simulink model "lhj_zero_optimize_2018a"  (R2018a)
settings: Solver=FixedStepDiscrete  StartTime=0.0  StopTime=0.2  FixedStep=Ts  RelTol=1e-4
InitFcn:
  | Ts=1e-6;
libraries: powerlib x17, simulink x2
settings Model: ExtModeTrigMode=oneshot  ExtModeArmWhenConnect=off  ExtModeAutoUpdateStatusClock=off  Creator=patrice  LastModifiedBy=chengqian
settings DataIOCC: SaveFormat=Array  SignalLoggingSaveFormat=ModelDataLogs  SignalLoggingName=sigsOut
settings OptimizationCC: BlockReduction=off  BooleanDataType=off  ExpressionDepthLimit=2147483647  InitFltsAndDblsToZero=on  LifeSpan=inf
settings DebuggingCC: SaveWithParameterizedLinksMsg=none  UnderspecifiedInitializationDetection=Classic  MergeDetectMultiDrivingBlocksExec=none  CheckExecutionContextPreStartOutputMsg=on  CheckExecutionContextRuntimeOutputMsg=on  SignalResolutionControl=TryResolveAllWithWarning  MultiTaskDSMMsg=warning  MultiTaskCondExecSysMsg=none  FcnCallInpInsideContextMsg=warning  UnconnectedLineMsg=none  StateNameClashWarn=warning  SFUnexpectedBacktrackingDiag=warning  SFNoUnconditionalDefaultTransitionDiag=warning  SFExecutionAtInitializationDiag=none
settings HardwareCC: ProdBitPerPointer=32  ProdBitPerSizeT=32  ProdBitPerPtrDiffT=32  ProdLargestAtomicFloat=None  ProdIntDivRoundTo=Undefined  ProdEndianess=Unspecified  ProdWordSize=32  ProdHWDeviceType=32-bit Generic  TargetUnknown=on
settings ModelReferenceCC: PropagateSignalLabelsOutOfModel=off
settings RTWCC: TemplateMakefile=grt_unix.tmf
settings CodeAppCC: StateflowObjectComments=on
settings GRTTargetCC: TargetFcnLib=ansi_tfl_tmw.mat  TargetLangStandard=C89/C90 (ANSI)  CombineOutputUpdateFcns=off  GRTInterface=on
settings ConfigComp: CovMetricSettings=dw  CovHtmlReporting=on  CovSaveCumulativeToWorkspaceVar=on  CovSaveSingleToWorkspaceVar=on  CovExternalEMLEnable=off

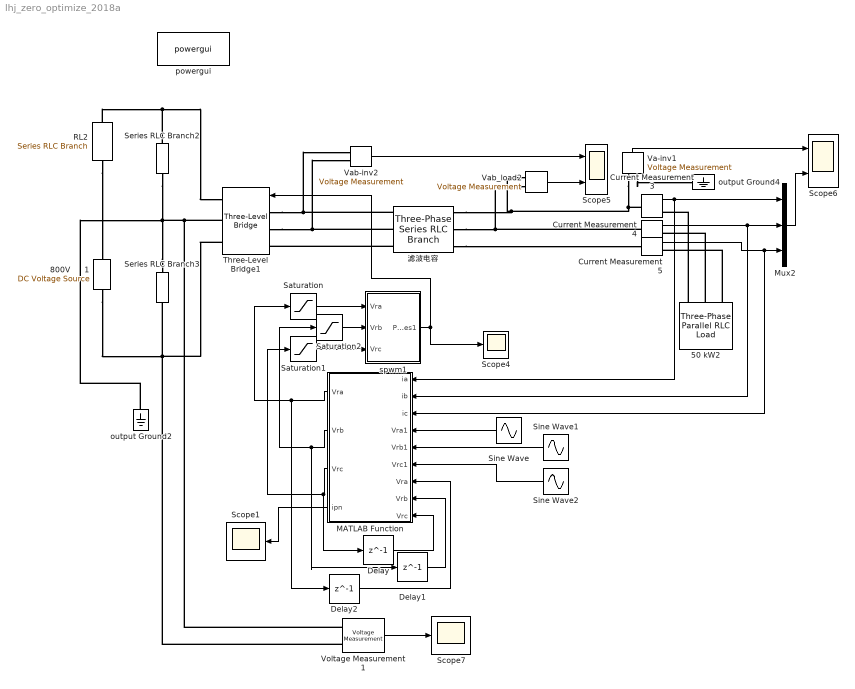
== system lhj_zero_optimize_2018a ==
  " 滤波电容" : powerlib/Elements/Three-Phase Series RLC Branch  LConnTagsString=A|B|C  RConnTagsString=A|B|C  BranchType=L  Resistance=0.1  Inductance=0.02  Capacitance=30e-3  Measurements=None
      settings: SourceProductName=Simscape Electrical
  50 kW2 : powerlib/Elements/Three-Phase Parallel RLC Load  LConnTagsString=A|B|C  Configuration=Y (grounded)  NominalVoltage=650  Vabc=[1e3 1e3 1e3]  Vabcp=[1e3 1e3 1e3]  NominalFrequency=50  UnbalancedPower=off  ActivePower=20000  InductivePower=0  CapacitivePower=0  Pabc=[10e3 9e3 11e3]  QLabc=[100 90 110]  QCabc=[100 90 110]  Pabcp=[10e3 9e3 11e3]  QLabcp=[100 90 110]  QCabcp=[100 90 110]  Measurements=Branch currents  LoadType=constant Z
      settings: SourceProductName=Simscape Electrical
  800V      1 : powerlib/Electrical Sources/DC Voltage Source  Description=source block  Amplitude=800  Measurements=None
      settings: AttributesFormatString=\n  SourceProductName=Simscape Electrical
  Current Measurement3 : powerlib/Measurements/Current Measurement  PhasorSimulation=off  OutputType=Complex  PSBequivalent=0
      settings: SourceProductName=Simscape Electrical
  Current Measurement4 : powerlib/Measurements/Current Measurement  PhasorSimulation=off  OutputType=Complex  PSBequivalent=0
      settings: SourceProductName=Simscape Electrical
  Current Measurement5 : powerlib/Measurements/Current Measurement  PhasorSimulation=off  OutputType=Complex  PSBequivalent=0
      settings: SourceProductName=Simscape Electrical
  Delay : Delay  DelayLength=1  InitialCondition=sin(2*pi*50 - 2/3*pi)
  Delay1 : Delay  DelayLength=1  InitialCondition=sin(2*pi*50 + 2/3*pi)
  Delay2 : Delay  DelayLength=1  InitialCondition=sin(2*pi*50)
  MATLAB Function : MATLAB Function  TreatAsAtomicUnit=on
  Mux2 : Mux  Inputs=3
  RL2 : powerlib/Elements/Series RLC Branch  LConnTagsString=__new0  RConnTagsString=__new0  BranchType=R  Resistance=1e-6  Inductance=1.0  SetiL0=off  InitialCurrent=0  Capacitance=1.0  Setx0=off  InitialVoltage=0  Measurements=None
      settings: SourceProductName=Simscape Electrical
  Saturation : Saturate  UpperLimit=1  LowerLimit=-1
  Saturation1 : Saturate  UpperLimit=1  LowerLimit=-1
  Saturation2 : Saturate  UpperLimit=1  LowerLimit=-1
  Scope1 : Scope
  Scope4 : Scope
  Scope5 : Scope  NumInputPorts=2
  Scope6 : Scope  NumInputPorts=2
  Scope7 : Scope
  Series RLC Branch2 : powerlib/Elements/Series RLC Branch  LConnTagsString=__new0  RConnTagsString=__new0  BranchType=C  Resistance=0  Inductance=0  SetiL0=off  InitialCurrent=0  Capacitance=7600e-6  Setx0=off  InitialVoltage=0  Measurements=None
      settings: SourceProductName=Simscape Electrical
  Series RLC Branch3 : powerlib/Elements/Series RLC Branch  LConnTagsString=__new0  RConnTagsString=__new0  BranchType=C  Resistance=0  Inductance=0  SetiL0=off  InitialCurrent=0  Capacitance=7600e-6  Setx0=off  InitialVoltage=0  Measurements=None
      settings: SourceProductName=Simscape Electrical
  Sine Wave : Sin  Frequency=2*pi*50  SampleTime=0
  Sine Wave1 : Sin  Frequency=2*pi*50  Phase=2/3*pi  SampleTime=0
  Sine Wave2 : Sin  Frequency=2*pi*50  Phase=-2/3*pi  SampleTime=0
  Three-Level Bridge1 : powerlib/Power Electronics/Three-Level Bridge  Arms=3  SnubberResistance=1e5  SbubberCapacitance=inf  Device=IGBT / Diodes  Ron=1e-6  ForwardVoltages="[  1  0.8]"  Measurements=None
      settings: SourceProductName=Simscape Electrical  SourceProductBaseCode=PS
  Va-inv1 : powerlib/Measurements/Voltage Measurement  Tag=PoWeRsYsTeMmEaSuReMeNt  PhasorSimulation=off  OutputType=Magnitude  PSBequivalent=0
      settings: SourceProductName=Simscape Electrical
  Vab-inv2 : powerlib/Measurements/Voltage Measurement  Tag=PoWeRsYsTeMmEaSuReMeNt  PhasorSimulation=off  OutputType=Magnitude  PSBequivalent=0
      settings: SourceProductName=Simscape Electrical
  Vab_load2 : powerlib/Measurements/Voltage Measurement  Tag=PoWeRsYsTeMmEaSuReMeNt  PhasorSimulation=off  OutputType=Magnitude  PSBequivalent=0
      settings: SourceProductName=Simscape Electrical
  Voltage Measurement1 : powerlib/Measurements/Voltage Measurement  PhasorSimulation=off  OutputType=Complex  PSBequivalent=0
      settings: SourceProductName=Simscape Electrical
  output Ground2 : powerlib/Elements/Ground  LConnTagsString=a
      settings: SourceProductName=Simscape Electrical
  output Ground4 : powerlib/Elements/Ground  LConnTagsString=a
      settings: SourceProductName=Simscape Electrical
  powergui : powerlib/powergui  SimulationMode=Discrete  SampleTime=Ts  frequency=60  Iterations=50  frequencyindice=0  Pbase=100e6  ErrMax=1e-4  UnitsV=kV  UnitsW=MW  buscounter=0  FunctionMessages=off  echomessages=on  EnableUseOfTLC=off  CurrentSourceSwitches=off  DisableSnubberDevices=off  DisableRonSwitches=off  DisableVfSwitches=off  DisplayEquations=off  SolverType=Tustin/Backward Euler (TBE)  Interpol=off  ExternalGateDelay=off  methode=off  Ts=0  x0status=blocks  SPID=off  SwTol=0  HookPort=off  RestoreLinks=warning  ResistiveCurrentMeasurement=off  Frange=[0:2:500]  Ylog=off  Xlog=on  ShowGrid=off  save=off  variable=ZData  structure=ScopeData3  ZoomFFT=off  StartTime=0.05-1/50  cycles=1  DisplayStyle=1  fundamental=50  FreqAxis=on  MaxFrequency=25000  frequencyindicesteady=1  RmsSteady=1  display=off
  spwm1 : Subsystem
  wires:
  Va-inv1/1 -> Scope6/1
  Vab_load2/1 -> Scope5/2
  Voltage Measurement1/1 -> Scope7/1
  Current Measurement3/1 -> MATLAB Function/1(ia), Mux2/1
  Mux2/1 -> Scope6/2
  Vab-inv2/1 -> Scope5/1
  Current Measurement4/1 -> MATLAB Function/2(ib), Mux2/2
  Current Measurement5/1 -> MATLAB Function/3(ic), Mux2/3
  spwm1/1(Pulses1) -> Scope4/1, Three-Level Bridge1/1
  MATLAB Function/1(Vra) -> Saturation/1, Delay2/1
  MATLAB Function/3(Vrc) -> Delay/1, Saturation1/1
  MATLAB Function/2(Vrb) -> Delay1/1, Saturation2/1
  Sine Wave1/1 -> MATLAB Function/5(Vrb1)
  Sine Wave/1 -> MATLAB Function/4(Vra1)
  Sine Wave2/1 -> MATLAB Function/6(Vrc1)
  Delay/1 -> MATLAB Function/9("Vrc ")
  Delay1/1 -> MATLAB Function/8("Vrb ")
  Delay2/1 -> MATLAB Function/7("Vra ")
  Saturation/1 -> spwm1/1(Vra)
  Saturation2/1 -> spwm1/2(Vrb)
  Saturation1/1 -> spwm1/3(Vrc)
  MATLAB Function/4(ipn) -> Scope1/1
  connections:
  Series RLC Branch3/LConn1 -- Voltage Measurement1/LConn1 -- Three-Level Bridge1/RConn2 -- Series RLC Branch2/RConn1 -- output Ground2/LConn1
  Three-Level Bridge1/LConn2 -- " 滤波电容"/LConn2 -- Vab-inv2/LConn2
  Vab_load2/LConn1 -- " 滤波电容"/RConn1 -- Current Measurement3/LConn1 -- Va-inv1/LConn1
  Current Measurement4/LConn1 -- " 滤波电容"/RConn2 -- Vab_load2/LConn2
  Three-Level Bridge1/LConn1 -- " 滤波电容"/LConn1 -- Vab-inv2/LConn1
  Voltage Measurement1/LConn2 -- Three-Level Bridge1/RConn3 -- 800V      1/LConn1 -- Series RLC Branch3/RConn1
  Series RLC Branch2/LConn1 -- Three-Level Bridge1/RConn1 -- RL2/LConn1
  50 kW2/LConn1 -- Current Measurement3/RConn1
  " 滤波电容"/LConn3 -- Three-Level Bridge1/LConn3
  50 kW2/LConn3 -- Current Measurement5/RConn1
  RL2/RConn1 -- 800V      1/RConn1
  " 滤波电容"/RConn3 -- Current Measurement5/LConn1
  Va-inv1/LConn2 -- output Ground4/LConn1
  50 kW2/LConn2 -- Current Measurement4/RConn1

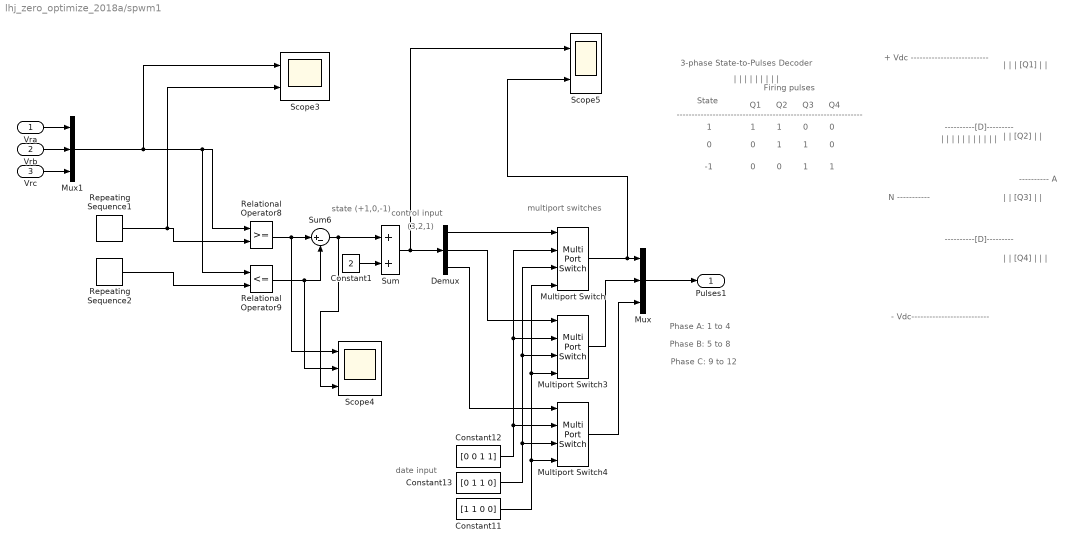
== system lhj_zero_optimize_2018a/spwm1 ==
  note: state
      | (+1,0,-1)
  note: Phase B: 5 to 8
  note: Phase A: 1 to 4
  note: Phase C: 9 to 12
  note: multiport switches
  note: date input
  note: control input
  note: (3,2,1)
  note: State
  note: 1
  note: Firing pulses
  note: 1
  note: 1
  note: 0
  note: 0
  note: Q1
  note: Q2
  note: Q3
  note: Q4
  note: 0
  note: 0
  note: 1
  note: 1
  note: 0
  note: -1
  note: 0
  note: 0
  note: 1
  note: 1
  note: |
      | |
      | |
      | |
      | |
      | |
      | |
      | |
      | |
  note: --------------------------------------------------------------
  note: 3-phase State-to-Pulses Decoder
  note: |
      | |
      | |
      | [Q1]
      | |
      | |
  note: |
      | |
      | [Q2]
      | |
      | |
  note: |
      | |
      | [Q3]
      | |
      | |
  note: |
      | |
      | [Q4]
      | |
      | |
      | |
  note: ----------[D]---------
  note: ----------[D]---------
  note: ---------- A
  note: |
      | |
      | |
      | |
      | |
      | |
      | |
      | |
      | |
      | |
      | |
  note: N -----------
  note: - Vdc--------------------------
  note: + Vdc --------------------------
  Vra : Inport
  Vrb : Inport  Port=2
  Vrc : Inport  Port=3
  Constant1 : Constant  Value=2
  Constant11 : Constant  Value=[1 1 0 0]
  Constant12 : Constant  Value=[0 0 1 1]
  Constant13 : Constant  Value=[0 1 1 0]
  Demux : Demux  Outputs=3
  Multiport Switch : MultiPortSwitch  InputSameDT=on
  Multiport Switch3 : MultiPortSwitch  InputSameDT=on
  Multiport Switch4 : MultiPortSwitch  InputSameDT=on
  Mux : Mux  Inputs=[4 4 4]
  Mux1 : Mux  Inputs=3
  Relational Operator8 : RelationalOperator  OutDataTypeStr=float('double')  RndMeth=Nearest  InputSameDT=on
  Relational Operator9 : RelationalOperator  Operator=<=  OutDataTypeStr=float('double')  RndMeth=Nearest  InputSameDT=on
  Repeating Sequence1 : simulink/Sources/Repeating Sequence  rep_seq_t=[0 0.0001 0.0002]  rep_seq_y=[0 1 0]
  Repeating Sequence2 : simulink/Sources/Repeating Sequence  rep_seq_t=[0 0.0001 0.0002]  rep_seq_y=[-1 0 -1]
  Scope3 : Scope  NumInputPorts=2
  Scope4 : Scope  NumInputPorts=3
  Scope5 : Scope  NumInputPorts=2
  Sum : Sum  SaturateOnIntegerOverflow=on  InputSameDT=on  OutDataTypeStr=Inherit: Same as first input
  Sum6 : Sum  Inputs=|+-  SaturateOnIntegerOverflow=on  InputSameDT=on  OutDataTypeStr=Inherit: Same as first input
  Pulses1 : Outport
  wires:
  Relational Operator9/1 -> Scope4/2, Sum6/2
  Mux/1 -> Pulses1/1
  Sum/1 -> Demux/1, Scope5/1
  Constant1/1 -> Sum/2
  Demux/1 -> Multiport Switch/1
  Demux/2 -> Multiport Switch3/1
  Demux/3 -> Multiport Switch4/1
  Constant12/1 -> Multiport Switch/2, Multiport Switch3/2, Multiport Switch4/2
  Constant13/1 -> Multiport Switch/3, Multiport Switch3/3, Multiport Switch4/3
  Constant11/1 -> Multiport Switch/4, Multiport Switch3/4, Multiport Switch4/4
  Multiport Switch/1 -> Scope5/2, Mux/1
  Multiport Switch3/1 -> Mux/2
  Multiport Switch4/1 -> Mux/3
  Repeating Sequence2/1 -> Relational Operator9/2
  Repeating Sequence1/1 -> Scope3/2, Relational Operator8/2
  Mux1/1 -> Scope3/1, Relational Operator9/1, Relational Operator8/1
  Relational Operator8/1 -> Scope4/1, Sum6/1
  Sum6/1 -> Scope4/3, Sum/1
  Vra/1 -> Mux1/1
  Vrb/1 -> Mux1/2
  Vrc/1 -> Mux1/3

== matlab function lhj_zero_optimize_2018a/MATLAB Function ==
  data: ia input; Vra output; ib input; ic input; Vra1 input; Vrb1 input; Vrc1 input; Vra input; Vrb input; Vrc input; Vrb output; Vrc output; ipn output
function [Vra,Vrb,Vrc,ipn] = fcn(ia,ib,ic,Vra1,Vrb1,Vrc1,Vra,Vrb,Vrc)

%%NPC型三电平变换器中点电压控制方法概述
Vo = -(sign(Vra)*Vra1*ia + sign(Vrb)*Vrb1*ib + sign(Vrc)*Vrc1*ic)/(sign(Vra)*ia + sign(Vrb)*ib + sign(Vrc)*ic);

ipn = -(sign(Vra)*Vra1*ia + sign(Vrb)*Vrb1*ib + sign(Vrc)*Vrc1*ic) - Vo*(sign(Vra)*ia + sign(Vrb)*ib + sign(Vrc)*ic);

Vra = Vra1 + Vo;
Vrb = Vrb1 + Vo;
Vrc = Vrc1 + Vo;
